simulink model "sync_simu"  (R2019b)
settings: Solver=VariableStepAuto  StartTime=0.0  StopTime=N_sim  RelTol=1e-3
InitFcn:
  | %% DSPBuilder Start
  | alt_dspbuilder_update_model(bdroot)
  | %% DSPBuilder End
  | 
  | sync_init
StartFcn:
  | %% DSPBuilder Start
  | alt_dspbuilder_hdlimport_prepare_for_simulation(bdroot)
  | %% DSPBuilder End
StopFcn:
  | sync_analysis
undefined symbols (not defined in the file or in its folder): __PRM__SERIALIZED__DATA__, SubsystemReferenceBlock
libraries: allblocks_alteradspbuilder2 x6, dspsrcs4 x2
settings Model: Creator=vboxuser  LastModifiedBy=vboxuser

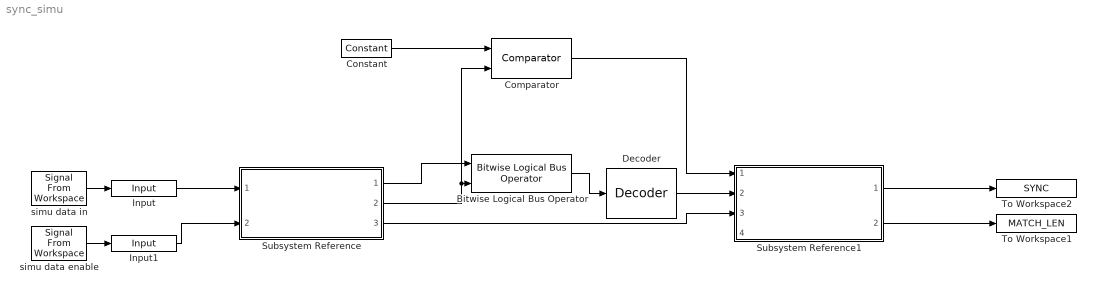
== system sync_simu ==
  Bitwise Logical Bus Operator : allblocks_alteradspbuilder2/Bitwise Logical Bus Operator  BusType=Unsigned Integer  bwl=8  bwr=0  LogicalOperator=XOR  pipeline_display=0
  Comparator : allblocks_alteradspbuilder2/Comparator  direction=a == b  pipeline_display=0  allowFloatingPointOverride=on  logOutputs=off  logFile=C:\Users\vboxuser\Documents\MATLAB\serializer\tb_sync_simu\sync%5Fsimu_Comparator.fixedpointlog
  Constant : allblocks_alteradspbuilder2/Constant  mask_cst=0x47  BusType=Unsigned Integer  bwl=8  bwr=0  roundMode=Truncate  satMode=Wrap  SpecifyClock=off  allowFloatingPointOverride=on  logOutputs=off  logFile=C:\Users\vboxuser\Documents\MATLAB\serializer\tb_sync_simu\sync%5Fsimu_Constant.fixedpointlog
  Decoder : allblocks_alteradspbuilder2/Decoder  BusType=Unsigned Integer  bwl=8  bwr=2  registered=off  pipeline_display=0  value=0xff
  Input : allblocks_alteradspbuilder2/Input  iofile=C:\Users\vboxuser\Documents\MATLAB\serializer\tb_sync_simu\sync%5Fsimu_Input.salt  BusType=Unsigned Integer  bwl=8  bwr=0  SpecifyClock=off  PORTTYPE=Input  externalType=Inferred  allowFloatingPointOverride=on  logOutputs=off
  Input1 : allblocks_alteradspbuilder2/Input  iofile=C:\Users\vboxuser\Documents\MATLAB\serializer\tb_sync_simu\sync%5Fsimu_Input1.salt  BusType=Unsigned Integer  bwl=8  bwr=0  SpecifyClock=off  PORTTYPE=Input  externalType=Inferred  allowFloatingPointOverride=on  logOutputs=off
  Subsystem Reference : Subsystem  BlockKeywords=__PRM__SERIALIZED__DATA__:SubsystemReferenceBlock  ReferencedSubsystem=deser  edge_triggered=off
  Subsystem Reference1 : Subsystem  BlockKeywords=__PRM__SERIALIZED__DATA__:SubsystemReferenceBlock  ReferencedSubsystem=matcher
  To Workspace1 : ToWorkspace  VariableName=MATCH_LEN  SampleTime=-1
      settings: Save2DSignal=2-D array (concatenate along first dimension)
  To Workspace2 : ToWorkspace  VariableName=SYNC  SampleTime=-1
      settings: Save2DSignal=2-D array (concatenate along first dimension)
  simu data enable : dspsrcs4/Signal From Workspace  X=data_en  Ts=1  nsamps=1  OutputAfterFinalValue=Setting to zero  ignoreOrWarnInputAndFrameLengths=off  OutputFrames=off
  simu data in : dspsrcs4/Signal From Workspace  X=data_in  Ts=1  nsamps=1  OutputAfterFinalValue=Setting to zero  ignoreOrWarnInputAndFrameLengths=off  OutputFrames=off
  wires:
  Subsystem Reference/2 -> Comparator/2, Bitwise Logical Bus Operator/2
  Constant/1 -> Comparator/1
  Subsystem Reference/3 -> Subsystem Reference1/3
  Comparator/1 -> Subsystem Reference1/1
  Subsystem Reference/1 -> Bitwise Logical Bus Operator/1
  Bitwise Logical Bus Operator/1 -> Decoder/1
  simu data in/1 -> Input/1
  simu data enable/1 -> Input1/1
  Decoder/1 -> Subsystem Reference1/2
  Input/1 -> Subsystem Reference/1
  Input1/1 -> Subsystem Reference/2
  Subsystem Reference1/1 -> To Workspace2/1
  Subsystem Reference1/2 -> To Workspace1/1
